simulink model "Avionics___Architecture_Model"  (R2022a)
settings: Solver=VariableStepAuto  StartTime=0.0  StopTime=10.0  RelTol=1e-3
settings Model: Creator=Kurt  LastModifiedBy=Kurt

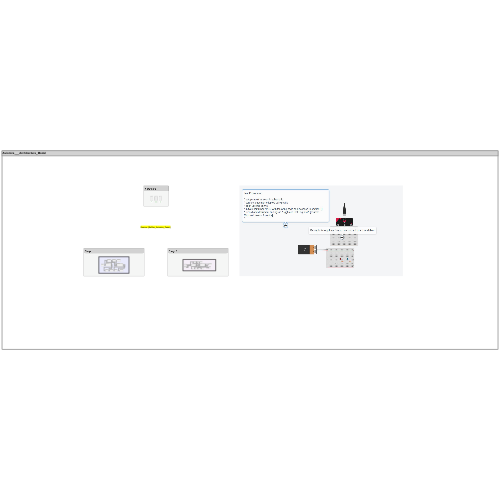
[thumbnail: Simulink's stored preview of the top-level diagram]
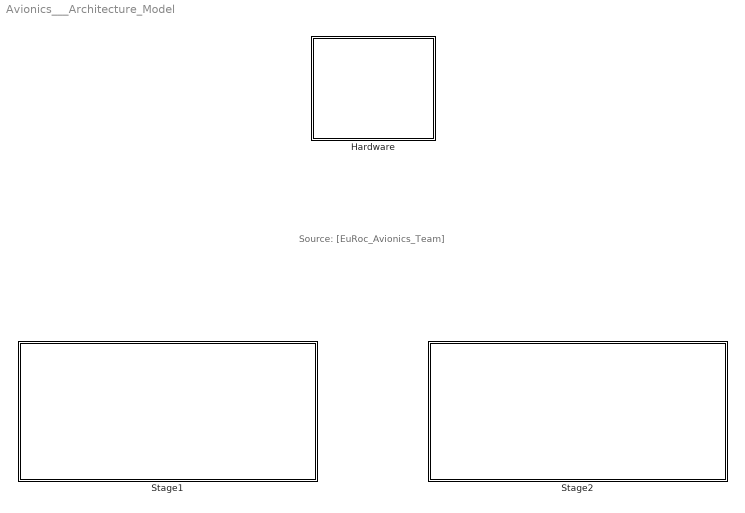
== system Avionics___Architecture_Model ==
  note: Source: [EuRoc_Avionics_Team]
  Hardware : Subsystem
      settings: PortSchema="{\"entries\":[{\"content\":{\"headerSize\":26,\"margin\":15,\"minimumSpacing\":25,\"sides\":[{\"content\":{\"connectorIds\":[]},\"type\":\"ConnectorPlacement.EquallySpacedRectSide\",\"uuid\":\"98d5147a-290e-4a67-98f4-450c53d1887a\"},{\"content\":{\"connectorIds\":[],\"side\":\"RIGHT\"},\"type\":\"ConnectorPlacement.EquallySpacedRectSide\",\"uuid\":\"a084b330-0c04-4420-9b8a-15d6db2d12b6\"},{\"content\":{\"connectorIds\":[],\"side\":\"TOP\"},\"type\":\"ConnectorPlacement.EquallySpacedRectSide\",\"uuid\":\"4cd23e2a-f423-4056-8b31-58661018ed01\"}]},\"type\":\"ConnectorPlacement.EquallySpacedConnector\",\"uuid\":\"58c578c1-1979-4184-bf96-9f147fef1420\"}],\"packageUris\":[\"http://schema.mathworks.com/mf0/Connector/R2020b\"],\"version\":\"1.0\"}"
  Stage1 : Subsystem
      settings: PortSchema="{\"entries\":[{\"content\":{\"headerSize\":26,\"margin\":15,\"minimumSpacing\":25,\"sides\":[{\"content\":{\"connectorIds\":[]},\"type\":\"ConnectorPlacement.EquallySpacedRectSide\",\"uuid\":\"98d5147a-290e-4a67-98f4-450c53d1887a\"},{\"content\":{\"connectorIds\":[],\"side\":\"RIGHT\"},\"type\":\"ConnectorPlacement.EquallySpacedRectSide\",\"uuid\":\"a084b330-0c04-4420-9b8a-15d6db2d12b6\"},{\"content\":{\"connectorIds\":[],\"side\":\"TOP\"},\"type\":\"ConnectorPlacement.EquallySpacedRectSide\",\"uuid\":\"4cd23e2a-f423-4056-8b31-58661018ed01\"}]},\"type\":\"ConnectorPlacement.EquallySpacedConnector\",\"uuid\":\"58c578c1-1979-4184-bf96-9f147fef1420\"}],\"packageUris\":[\"http://schema.mathworks.com/mf0/Connector/R2020b\"],\"version\":\"1.0\"}"
  Stage2 : Subsystem
      settings: PortSchema="{\"entries\":[{\"content\":{\"headerSize\":26,\"margin\":15,\"minimumSpacing\":25,\"sides\":[{\"content\":{\"connectorIds\":[]},\"type\":\"ConnectorPlacement.EquallySpacedRectSide\",\"uuid\":\"98d5147a-290e-4a67-98f4-450c53d1887a\"},{\"content\":{\"connectorIds\":[],\"side\":\"RIGHT\"},\"type\":\"ConnectorPlacement.EquallySpacedRectSide\",\"uuid\":\"a084b330-0c04-4420-9b8a-15d6db2d12b6\"},{\"content\":{\"connectorIds\":[],\"side\":\"TOP\"},\"type\":\"ConnectorPlacement.EquallySpacedRectSide\",\"uuid\":\"4cd23e2a-f423-4056-8b31-58661018ed01\"}]},\"type\":\"ConnectorPlacement.EquallySpacedConnector\",\"uuid\":\"58c578c1-1979-4184-bf96-9f147fef1420\"}],\"packageUris\":[\"http://schema.mathworks.com/mf0/Connector/R2020b\"],\"version\":\"1.0\"}"

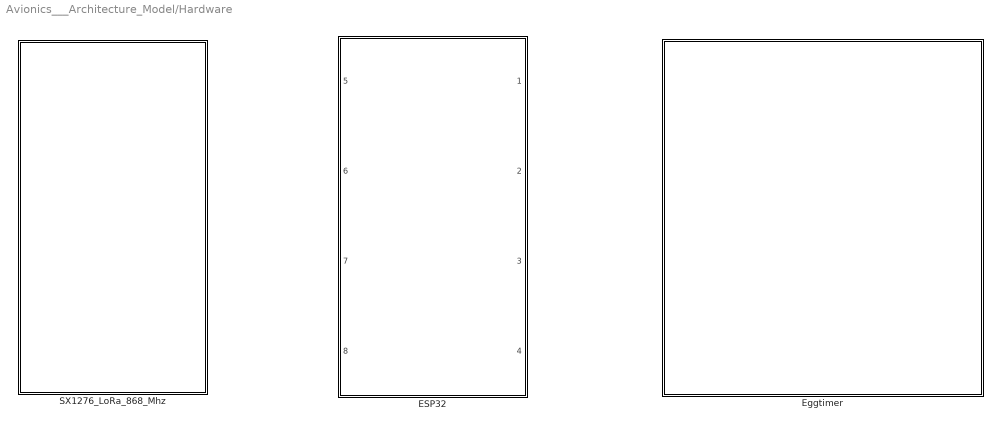
== system Avionics___Architecture_Model/Hardware ==
  ESP32 : Subsystem
      settings: PortSchema="{\"entries\":[{\"content\":{\"headerSize\":26,\"margin\":15,\"minimumSpacing\":25,\"sides\":[{\"content\":{\"connectorIds\":[\"In1\",\"In2\",\"In3\",\"In4\"]},\"type\":\"ConnectorPlacement.EquallySpacedRectSide\",\"uuid\":\"98d5147a-290e-4a67-98f4-450c53d1887a\"},{\"content\":{\"connectorIds\":[\"Out1\",\"Out2\",\"Out3\",\"Out4\"],\"side\":\"RIGHT\"},\"type\":\"ConnectorPlacement.EquallySpacedRectSide\",\"uuid\":\"a084b330-0c04-4420-9b8a-15d6db2d12b6\"},{\"content\":{\"connectorIds\":[],\"side\":\"TOP\"},\"type\":\"ConnectorPlacement.EquallySpacedRectSide\",\"uuid\":\"4cd23e2a-f423-4056-8b31-58661018ed01\"}]},\"type\":\"ConnectorPlacement.EquallySpacedConnector\",\"uuid\":\"58c578c1-1979-4184-bf96-9f147fef1420\"}],\"packageUris\":[\"http://schema.mathworks.com/mf0/Connector/R2020b\"],\"version\":\"1.0\"}"
  Eggtimer : Subsystem
      settings: PortSchema="{\"entries\":[{\"content\":{\"headerSize\":26,\"margin\":15,\"minimumSpacing\":25,\"sides\":[{\"content\":{\"connectorIds\":[\"LConn1\",\"LConn2\"]},\"type\":\"ConnectorPlacement.EquallySpacedRectSide\",\"uuid\":\"98d5147a-290e-4a67-98f4-450c53d1887a\"},{\"content\":{\"connectorIds\":[\"RConn1\",\"RConn2\",\"RConn3\",\"RConn4\"],\"side\":\"RIGHT\"},\"type\":\"ConnectorPlacement.EquallySpacedRectSide\",\"uuid\":\"a084b330-0c04-4420-9b8a-15d6db2d12b6\"},{\"content\":{\"connectorIds\":[\"LConn3\",\"LConn4\",\"LConn5\",\"LConn6\",\"LConn7\",\"LConn8\",\"LConn9\",\"LConn10\"],\"side\":\"TOP\"},\"type\":\"ConnectorPlacement.EquallySpacedRectSide\",\"uuid\":\"4cd23e2a-f423-4056-8b31-58661018ed01\"},{\"content\":{\"connectorIds\":[\"RConn5\",\"RConn6\",\"RConn7\",\"RConn8\",\"RConn9\",\"RConn10\"],\"side\":\"BOTTOM\"},\"type\":\"ConnectorPlacement.EquallySpacedRectSide\",\"uuid\":\"c712a256-adbb-4d26-ab18-9b9cb2ad7b77\"}]},\"type\":\"ConnectorPlacement.EquallySpacedConnector\",\"uuid\":\"58c578c1-1979-4184-bf96-9f147fef1420\"}],\"packageUris\":[\"http://schema.mathworks.com/mf0/Connector/R2020b\"],\"version\":\"1.0\"}"
  SX1276_LoRa_868_Mhz : Subsystem
      settings: PortSchema="{\"entries\":[{\"content\":{\"headerSize\":26,\"margin\":15,\"minimumSpacing\":25,\"sides\":[{\"content\":{\"connectorIds\":[]},\"type\":\"ConnectorPlacement.EquallySpacedRectSide\",\"uuid\":\"98d5147a-290e-4a67-98f4-450c53d1887a\"},{\"content\":{\"connectorIds\":[],\"side\":\"RIGHT\"},\"type\":\"ConnectorPlacement.EquallySpacedRectSide\",\"uuid\":\"a084b330-0c04-4420-9b8a-15d6db2d12b6\"},{\"content\":{\"connectorIds\":[],\"side\":\"TOP\"},\"type\":\"ConnectorPlacement.EquallySpacedRectSide\",\"uuid\":\"4cd23e2a-f423-4056-8b31-58661018ed01\"}]},\"type\":\"ConnectorPlacement.EquallySpacedConnector\",\"uuid\":\"58c578c1-1979-4184-bf96-9f147fef1420\"}],\"packageUris\":[\"http://schema.mathworks.com/mf0/Connector/R2020b\"],\"version\":\"1.0\"}"

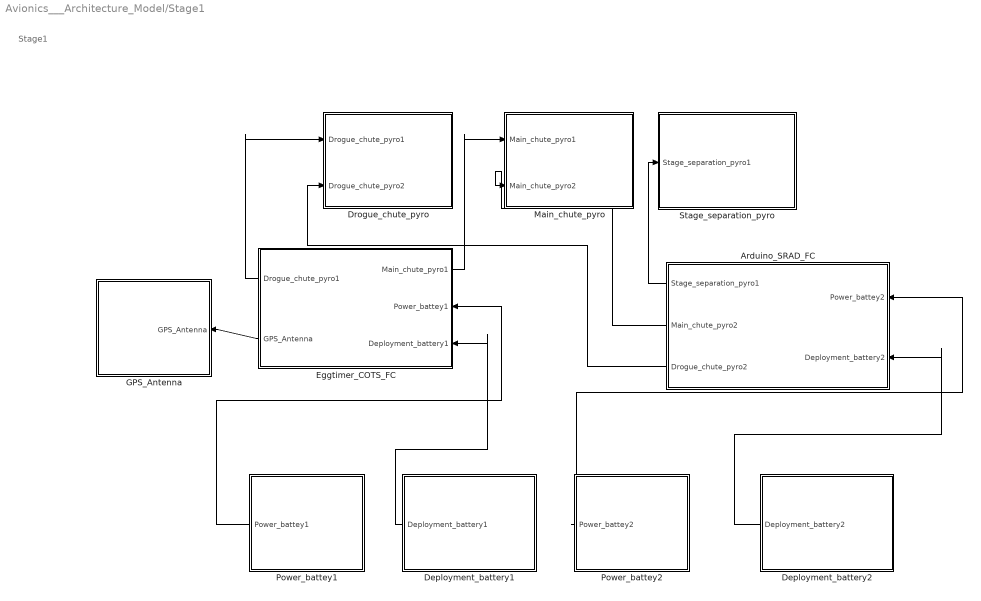
== system Avionics___Architecture_Model/Stage1 ==
  note: Stage1
  Arduino_SRAD_FC : Subsystem
      settings: PortSchema="{\"entries\":[{\"content\":{\"headerSize\":26,\"margin\":15,\"minimumSpacing\":25,\"sides\":[{\"content\":{\"connectorIds\":[\"Out1\",\"Out2\",\"Out3\"]},\"type\":\"ConnectorPlacement.EquallySpacedRectSide\",\"uuid\":\"98d5147a-290e-4a67-98f4-450c53d1887a\"},{\"content\":{\"connectorIds\":[\"In2\",\"In1\"],\"side\":\"RIGHT\"},\"type\":\"ConnectorPlacement.EquallySpacedRectSide\",\"uuid\":\"a084b330-0c04-4420-9b8a-15d6db2d12b6\"},{\"content\":{\"connectorIds\":[],\"side\":\"TOP\"},\"type\":\"ConnectorPlacement.EquallySpacedRectSide\",\"uuid\":\"4cd23e2a-f423-4056-8b31-58661018ed01\"},{\"content\":{\"connectorIds\":[],\"side\":\"BOTTOM\"},\"type\":\"ConnectorPlacement.EquallySpacedRectSide\",\"uuid\":\"eb863bb0-7cf9-4bf2-bc0b-ec6aafea4d0a\"}]},\"type\":\"ConnectorPlacement.EquallySpacedConnector\",\"uuid\":\"58c578c1-1979-4184-bf96-9f147fef1420\"}],\"packageUris\":[\"http://schema.mathworks.com/mf0/Connector/R2020b\"],\"version\":\"1.0\"}"
  Deployment_battery1 : Subsystem
      settings: PortSchema="{\"entries\":[{\"content\":{\"headerSize\":26,\"margin\":15,\"minimumSpacing\":25,\"sides\":[{\"content\":{\"connectorIds\":[\"Out1\"]},\"type\":\"ConnectorPlacement.EquallySpacedRectSide\",\"uuid\":\"98d5147a-290e-4a67-98f4-450c53d1887a\"},{\"content\":{\"connectorIds\":[],\"side\":\"RIGHT\"},\"type\":\"ConnectorPlacement.EquallySpacedRectSide\",\"uuid\":\"a084b330-0c04-4420-9b8a-15d6db2d12b6\"},{\"content\":{\"connectorIds\":[],\"side\":\"TOP\"},\"type\":\"ConnectorPlacement.EquallySpacedRectSide\",\"uuid\":\"4cd23e2a-f423-4056-8b31-58661018ed01\"}]},\"type\":\"ConnectorPlacement.EquallySpacedConnector\",\"uuid\":\"58c578c1-1979-4184-bf96-9f147fef1420\"}],\"packageUris\":[\"http://schema.mathworks.com/mf0/Connector/R2020b\"],\"version\":\"1.0\"}"
  Deployment_battery2 : Subsystem
      settings: PortSchema="{\"entries\":[{\"content\":{\"headerSize\":26,\"margin\":15,\"minimumSpacing\":25,\"sides\":[{\"content\":{\"connectorIds\":[\"Out1\"]},\"type\":\"ConnectorPlacement.EquallySpacedRectSide\",\"uuid\":\"98d5147a-290e-4a67-98f4-450c53d1887a\"},{\"content\":{\"connectorIds\":[],\"side\":\"RIGHT\"},\"type\":\"ConnectorPlacement.EquallySpacedRectSide\",\"uuid\":\"a084b330-0c04-4420-9b8a-15d6db2d12b6\"},{\"content\":{\"connectorIds\":[],\"side\":\"TOP\"},\"type\":\"ConnectorPlacement.EquallySpacedRectSide\",\"uuid\":\"4cd23e2a-f423-4056-8b31-58661018ed01\"}]},\"type\":\"ConnectorPlacement.EquallySpacedConnector\",\"uuid\":\"58c578c1-1979-4184-bf96-9f147fef1420\"}],\"packageUris\":[\"http://schema.mathworks.com/mf0/Connector/R2020b\"],\"version\":\"1.0\"}"
  Drogue_chute_pyro : Subsystem  Description=Reference: [Preliminary_CDR, CranSEDS,avionics team]
      settings: PortSchema="{\"entries\":[{\"content\":{\"headerSize\":26,\"margin\":15,\"minimumSpacing\":25,\"sides\":[{\"content\":{\"connectorIds\":[\"In1\",\"In2\"]},\"type\":\"ConnectorPlacement.EquallySpacedRectSide\",\"uuid\":\"98d5147a-290e-4a67-98f4-450c53d1887a\"},{\"content\":{\"connectorIds\":[],\"side\":\"RIGHT\"},\"type\":\"ConnectorPlacement.EquallySpacedRectSide\",\"uuid\":\"a084b330-0c04-4420-9b8a-15d6db2d12b6\"},{\"content\":{\"connectorIds\":[],\"side\":\"TOP\"},\"type\":\"ConnectorPlacement.EquallySpacedRectSide\",\"uuid\":\"4cd23e2a-f423-4056-8b31-58661018ed01\"}]},\"type\":\"ConnectorPlacement.EquallySpacedConnector\",\"uuid\":\"58c578c1-1979-4184-bf96-9f147fef1420\"}],\"packageUris\":[\"http://schema.mathworks.com/mf0/Connector/R2020b\"],\"version\":\"1.0\"}"
  Eggtimer_COTS_FC : Subsystem
      settings: PortSchema="{\"entries\":[{\"content\":{\"headerSize\":26,\"margin\":15,\"minimumSpacing\":25,\"sides\":[{\"content\":{\"connectorIds\":[\"Out2\",\"Out3\"]},\"type\":\"ConnectorPlacement.EquallySpacedRectSide\",\"uuid\":\"98d5147a-290e-4a67-98f4-450c53d1887a\"},{\"content\":{\"connectorIds\":[\"Out1\",\"In1\",\"In2\"],\"side\":\"RIGHT\"},\"type\":\"ConnectorPlacement.EquallySpacedRectSide\",\"uuid\":\"a084b330-0c04-4420-9b8a-15d6db2d12b6\"},{\"content\":{\"connectorIds\":[],\"side\":\"TOP\"},\"type\":\"ConnectorPlacement.EquallySpacedRectSide\",\"uuid\":\"4cd23e2a-f423-4056-8b31-58661018ed01\"}]},\"type\":\"ConnectorPlacement.EquallySpacedConnector\",\"uuid\":\"58c578c1-1979-4184-bf96-9f147fef1420\"}],\"packageUris\":[\"http://schema.mathworks.com/mf0/Connector/R2020b\"],\"version\":\"1.0\"}"
  GPS_Antenna : Subsystem
      settings: PortSchema="{\"entries\":[{\"content\":{\"headerSize\":26,\"margin\":15,\"minimumSpacing\":25,\"sides\":[{\"content\":{\"connectorIds\":[]},\"type\":\"ConnectorPlacement.EquallySpacedRectSide\",\"uuid\":\"98d5147a-290e-4a67-98f4-450c53d1887a\"},{\"content\":{\"connectorIds\":[\"In1\"],\"side\":\"RIGHT\"},\"type\":\"ConnectorPlacement.EquallySpacedRectSide\",\"uuid\":\"a084b330-0c04-4420-9b8a-15d6db2d12b6\"},{\"content\":{\"connectorIds\":[],\"side\":\"TOP\"},\"type\":\"ConnectorPlacement.EquallySpacedRectSide\",\"uuid\":\"4cd23e2a-f423-4056-8b31-58661018ed01\"}]},\"type\":\"ConnectorPlacement.EquallySpacedConnector\",\"uuid\":\"58c578c1-1979-4184-bf96-9f147fef1420\"}],\"packageUris\":[\"http://schema.mathworks.com/mf0/Connector/R2020b\"],\"version\":\"1.0\"}"
  Main_chute_pyro : Subsystem
      settings: PortSchema="{\"entries\":[{\"content\":{\"headerSize\":26,\"margin\":15,\"minimumSpacing\":25,\"sides\":[{\"content\":{\"connectorIds\":[\"In1\",\"In2\"]},\"type\":\"ConnectorPlacement.EquallySpacedRectSide\",\"uuid\":\"98d5147a-290e-4a67-98f4-450c53d1887a\"},{\"content\":{\"connectorIds\":[],\"side\":\"RIGHT\"},\"type\":\"ConnectorPlacement.EquallySpacedRectSide\",\"uuid\":\"a084b330-0c04-4420-9b8a-15d6db2d12b6\"},{\"content\":{\"connectorIds\":[],\"side\":\"TOP\"},\"type\":\"ConnectorPlacement.EquallySpacedRectSide\",\"uuid\":\"4cd23e2a-f423-4056-8b31-58661018ed01\"}]},\"type\":\"ConnectorPlacement.EquallySpacedConnector\",\"uuid\":\"58c578c1-1979-4184-bf96-9f147fef1420\"}],\"packageUris\":[\"http://schema.mathworks.com/mf0/Connector/R2020b\"],\"version\":\"1.0\"}"
  Power_battey1 : Subsystem
      settings: PortSchema="{\"entries\":[{\"content\":{\"headerSize\":26,\"margin\":15,\"minimumSpacing\":25,\"sides\":[{\"content\":{\"connectorIds\":[\"Out1\"]},\"type\":\"ConnectorPlacement.EquallySpacedRectSide\",\"uuid\":\"98d5147a-290e-4a67-98f4-450c53d1887a\"},{\"content\":{\"connectorIds\":[],\"side\":\"RIGHT\"},\"type\":\"ConnectorPlacement.EquallySpacedRectSide\",\"uuid\":\"a084b330-0c04-4420-9b8a-15d6db2d12b6\"},{\"content\":{\"connectorIds\":[],\"side\":\"TOP\"},\"type\":\"ConnectorPlacement.EquallySpacedRectSide\",\"uuid\":\"4cd23e2a-f423-4056-8b31-58661018ed01\"}]},\"type\":\"ConnectorPlacement.EquallySpacedConnector\",\"uuid\":\"58c578c1-1979-4184-bf96-9f147fef1420\"}],\"packageUris\":[\"http://schema.mathworks.com/mf0/Connector/R2020b\"],\"version\":\"1.0\"}"
  Power_battey2 : Subsystem
      settings: PortSchema="{\"entries\":[{\"content\":{\"headerSize\":26,\"margin\":15,\"minimumSpacing\":25,\"sides\":[{\"content\":{\"connectorIds\":[\"Out1\"]},\"type\":\"ConnectorPlacement.EquallySpacedRectSide\",\"uuid\":\"98d5147a-290e-4a67-98f4-450c53d1887a\"},{\"content\":{\"connectorIds\":[],\"side\":\"RIGHT\"},\"type\":\"ConnectorPlacement.EquallySpacedRectSide\",\"uuid\":\"a084b330-0c04-4420-9b8a-15d6db2d12b6\"},{\"content\":{\"connectorIds\":[],\"side\":\"TOP\"},\"type\":\"ConnectorPlacement.EquallySpacedRectSide\",\"uuid\":\"4cd23e2a-f423-4056-8b31-58661018ed01\"}]},\"type\":\"ConnectorPlacement.EquallySpacedConnector\",\"uuid\":\"58c578c1-1979-4184-bf96-9f147fef1420\"}],\"packageUris\":[\"http://schema.mathworks.com/mf0/Connector/R2020b\"],\"version\":\"1.0\"}"
  Stage_separation_pyro : Subsystem
      settings: PortSchema="{\"entries\":[{\"content\":{\"headerSize\":26,\"margin\":15,\"minimumSpacing\":25,\"sides\":[{\"content\":{\"connectorIds\":[\"In1\"]},\"type\":\"ConnectorPlacement.EquallySpacedRectSide\",\"uuid\":\"98d5147a-290e-4a67-98f4-450c53d1887a\"},{\"content\":{\"connectorIds\":[],\"side\":\"RIGHT\"},\"type\":\"ConnectorPlacement.EquallySpacedRectSide\",\"uuid\":\"a084b330-0c04-4420-9b8a-15d6db2d12b6\"},{\"content\":{\"connectorIds\":[],\"side\":\"TOP\"},\"type\":\"ConnectorPlacement.EquallySpacedRectSide\",\"uuid\":\"4cd23e2a-f423-4056-8b31-58661018ed01\"}]},\"type\":\"ConnectorPlacement.EquallySpacedConnector\",\"uuid\":\"58c578c1-1979-4184-bf96-9f147fef1420\"}],\"packageUris\":[\"http://schema.mathworks.com/mf0/Connector/R2020b\"],\"version\":\"1.0\"}"
  wires:
  Arduino_SRAD_FC/3(Drogue_chute_pyro2) -> Drogue_chute_pyro/2(Drogue_chute_pyro2)
  Deployment_battery1/1(Deployment_battery1) -> Eggtimer_COTS_FC/2(Deployment_battery1)
  Eggtimer_COTS_FC/2(Drogue_chute_pyro1) -> Drogue_chute_pyro/1(Drogue_chute_pyro1)
  Arduino_SRAD_FC/2(Main_chute_pyro2) -> Main_chute_pyro/2(Main_chute_pyro2)
  Eggtimer_COTS_FC/3(GPS_Antenna) -> GPS_Antenna/1(GPS_Antenna)
  Power_battey1/1(Power_battey1) -> Eggtimer_COTS_FC/1(Power_battey1)
  Eggtimer_COTS_FC/1(Main_chute_pyro1) -> Main_chute_pyro/1(Main_chute_pyro1)
  Arduino_SRAD_FC/1(Stage_separation_pyro1) -> Stage_separation_pyro/1(Stage_separation_pyro1)
  Deployment_battery2/1(Deployment_battery2) -> Arduino_SRAD_FC/1(Deployment_battery2)
  Power_battey2/1(Power_battey2) -> Arduino_SRAD_FC/2(Power_battey2)

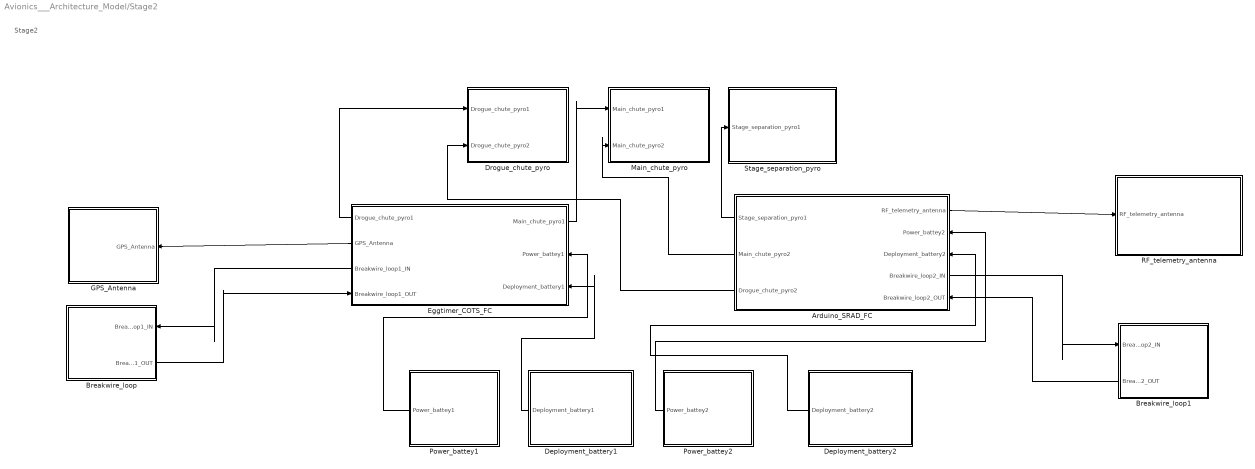
== system Avionics___Architecture_Model/Stage2 ==
  note: Stage2
  Arduino_SRAD_FC : Subsystem
      settings: PortSchema="{\"entries\":[{\"content\":{\"headerSize\":26,\"margin\":15,\"minimumSpacing\":25,\"sides\":[{\"content\":{\"connectorIds\":[\"Out3\",\"Out4\",\"Out5\"]},\"type\":\"ConnectorPlacement.EquallySpacedRectSide\",\"uuid\":\"98d5147a-290e-4a67-98f4-450c53d1887a\"},{\"content\":{\"connectorIds\":[\"Out1\",\"In2\",\"In1\",\"Out2\",\"In3\"],\"side\":\"RIGHT\"},\"type\":\"ConnectorPlacement.EquallySpacedRectSide\",\"uuid\":\"a084b330-0c04-4420-9b8a-15d6db2d12b6\"},{\"content\":{\"connectorIds\":[],\"side\":\"TOP\"},\"type\":\"ConnectorPlacement.EquallySpacedRectSide\",\"uuid\":\"4cd23e2a-f423-4056-8b31-58661018ed01\"},{\"content\":{\"connectorIds\":[],\"side\":\"BOTTOM\"},\"type\":\"ConnectorPlacement.EquallySpacedRectSide\",\"uuid\":\"eb863bb0-7cf9-4bf2-bc0b-ec6aafea4d0a\"}]},\"type\":\"ConnectorPlacement.EquallySpacedConnector\",\"uuid\":\"58c578c1-1979-4184-bf96-9f147fef1420\"}],\"packageUris\":[\"http://schema.mathworks.com/mf0/Connector/R2020b\"],\"version\":\"1.0\"}"
  Breakwire_loop : Subsystem
      settings: PortSchema="{\"entries\":[{\"content\":{\"headerSize\":26,\"margin\":15,\"minimumSpacing\":25,\"sides\":[{\"content\":{\"connectorIds\":[]},\"type\":\"ConnectorPlacement.EquallySpacedRectSide\",\"uuid\":\"98d5147a-290e-4a67-98f4-450c53d1887a\"},{\"content\":{\"connectorIds\":[\"In1\",\"Out1\"],\"side\":\"RIGHT\"},\"type\":\"ConnectorPlacement.EquallySpacedRectSide\",\"uuid\":\"a084b330-0c04-4420-9b8a-15d6db2d12b6\"},{\"content\":{\"connectorIds\":[],\"side\":\"TOP\"},\"type\":\"ConnectorPlacement.EquallySpacedRectSide\",\"uuid\":\"4cd23e2a-f423-4056-8b31-58661018ed01\"}]},\"type\":\"ConnectorPlacement.EquallySpacedConnector\",\"uuid\":\"58c578c1-1979-4184-bf96-9f147fef1420\"}],\"packageUris\":[\"http://schema.mathworks.com/mf0/Connector/R2020b\"],\"version\":\"1.0\"}"
  Breakwire_loop1 : Subsystem
      settings: PortSchema="{\"entries\":[{\"content\":{\"headerSize\":26,\"margin\":15,\"minimumSpacing\":25,\"sides\":[{\"content\":{\"connectorIds\":[\"In1\",\"Out1\"]},\"type\":\"ConnectorPlacement.EquallySpacedRectSide\",\"uuid\":\"98d5147a-290e-4a67-98f4-450c53d1887a\"},{\"content\":{\"connectorIds\":[],\"side\":\"RIGHT\"},\"type\":\"ConnectorPlacement.EquallySpacedRectSide\",\"uuid\":\"a084b330-0c04-4420-9b8a-15d6db2d12b6\"},{\"content\":{\"connectorIds\":[],\"side\":\"TOP\"},\"type\":\"ConnectorPlacement.EquallySpacedRectSide\",\"uuid\":\"4cd23e2a-f423-4056-8b31-58661018ed01\"}]},\"type\":\"ConnectorPlacement.EquallySpacedConnector\",\"uuid\":\"58c578c1-1979-4184-bf96-9f147fef1420\"}],\"packageUris\":[\"http://schema.mathworks.com/mf0/Connector/R2020b\"],\"version\":\"1.0\"}"
  Deployment_battery1 : Subsystem
      settings: PortSchema="{\"entries\":[{\"content\":{\"headerSize\":26,\"margin\":15,\"minimumSpacing\":25,\"sides\":[{\"content\":{\"connectorIds\":[\"Out1\"]},\"type\":\"ConnectorPlacement.EquallySpacedRectSide\",\"uuid\":\"98d5147a-290e-4a67-98f4-450c53d1887a\"},{\"content\":{\"connectorIds\":[],\"side\":\"RIGHT\"},\"type\":\"ConnectorPlacement.EquallySpacedRectSide\",\"uuid\":\"a084b330-0c04-4420-9b8a-15d6db2d12b6\"},{\"content\":{\"connectorIds\":[],\"side\":\"TOP\"},\"type\":\"ConnectorPlacement.EquallySpacedRectSide\",\"uuid\":\"4cd23e2a-f423-4056-8b31-58661018ed01\"}]},\"type\":\"ConnectorPlacement.EquallySpacedConnector\",\"uuid\":\"58c578c1-1979-4184-bf96-9f147fef1420\"}],\"packageUris\":[\"http://schema.mathworks.com/mf0/Connector/R2020b\"],\"version\":\"1.0\"}"
  Deployment_battery2 : Subsystem
      settings: PortSchema="{\"entries\":[{\"content\":{\"headerSize\":26,\"margin\":15,\"minimumSpacing\":25,\"sides\":[{\"content\":{\"connectorIds\":[\"Out1\"]},\"type\":\"ConnectorPlacement.EquallySpacedRectSide\",\"uuid\":\"98d5147a-290e-4a67-98f4-450c53d1887a\"},{\"content\":{\"connectorIds\":[],\"side\":\"RIGHT\"},\"type\":\"ConnectorPlacement.EquallySpacedRectSide\",\"uuid\":\"a084b330-0c04-4420-9b8a-15d6db2d12b6\"},{\"content\":{\"connectorIds\":[],\"side\":\"TOP\"},\"type\":\"ConnectorPlacement.EquallySpacedRectSide\",\"uuid\":\"4cd23e2a-f423-4056-8b31-58661018ed01\"}]},\"type\":\"ConnectorPlacement.EquallySpacedConnector\",\"uuid\":\"58c578c1-1979-4184-bf96-9f147fef1420\"}],\"packageUris\":[\"http://schema.mathworks.com/mf0/Connector/R2020b\"],\"version\":\"1.0\"}"
  Drogue_chute_pyro : Subsystem  Description=Reference: [Preliminary_CDR, CranSEDS,avionics team]
      settings: PortSchema="{\"entries\":[{\"content\":{\"headerSize\":26,\"margin\":15,\"minimumSpacing\":25,\"sides\":[{\"content\":{\"connectorIds\":[\"In1\",\"In2\"]},\"type\":\"ConnectorPlacement.EquallySpacedRectSide\",\"uuid\":\"98d5147a-290e-4a67-98f4-450c53d1887a\"},{\"content\":{\"connectorIds\":[],\"side\":\"RIGHT\"},\"type\":\"ConnectorPlacement.EquallySpacedRectSide\",\"uuid\":\"a084b330-0c04-4420-9b8a-15d6db2d12b6\"},{\"content\":{\"connectorIds\":[],\"side\":\"TOP\"},\"type\":\"ConnectorPlacement.EquallySpacedRectSide\",\"uuid\":\"4cd23e2a-f423-4056-8b31-58661018ed01\"}]},\"type\":\"ConnectorPlacement.EquallySpacedConnector\",\"uuid\":\"58c578c1-1979-4184-bf96-9f147fef1420\"}],\"packageUris\":[\"http://schema.mathworks.com/mf0/Connector/R2020b\"],\"version\":\"1.0\"}"
  Eggtimer_COTS_FC : Subsystem
      settings: PortSchema="{\"entries\":[{\"content\":{\"headerSize\":26,\"margin\":15,\"minimumSpacing\":25,\"sides\":[{\"content\":{\"connectorIds\":[\"Out2\",\"Out4\",\"Out3\",\"In1\"]},\"type\":\"ConnectorPlacement.EquallySpacedRectSide\",\"uuid\":\"98d5147a-290e-4a67-98f4-450c53d1887a\"},{\"content\":{\"connectorIds\":[\"Out1\",\"In2\",\"In3\"],\"side\":\"RIGHT\"},\"type\":\"ConnectorPlacement.EquallySpacedRectSide\",\"uuid\":\"a084b330-0c04-4420-9b8a-15d6db2d12b6\"},{\"content\":{\"connectorIds\":[],\"side\":\"TOP\"},\"type\":\"ConnectorPlacement.EquallySpacedRectSide\",\"uuid\":\"4cd23e2a-f423-4056-8b31-58661018ed01\"}]},\"type\":\"ConnectorPlacement.EquallySpacedConnector\",\"uuid\":\"58c578c1-1979-4184-bf96-9f147fef1420\"}],\"packageUris\":[\"http://schema.mathworks.com/mf0/Connector/R2020b\"],\"version\":\"1.0\"}"
  GPS_Antenna : Subsystem
      settings: PortSchema="{\"entries\":[{\"content\":{\"headerSize\":26,\"margin\":15,\"minimumSpacing\":25,\"sides\":[{\"content\":{\"connectorIds\":[]},\"type\":\"ConnectorPlacement.EquallySpacedRectSide\",\"uuid\":\"98d5147a-290e-4a67-98f4-450c53d1887a\"},{\"content\":{\"connectorIds\":[\"In1\"],\"side\":\"RIGHT\"},\"type\":\"ConnectorPlacement.EquallySpacedRectSide\",\"uuid\":\"a084b330-0c04-4420-9b8a-15d6db2d12b6\"},{\"content\":{\"connectorIds\":[],\"side\":\"TOP\"},\"type\":\"ConnectorPlacement.EquallySpacedRectSide\",\"uuid\":\"4cd23e2a-f423-4056-8b31-58661018ed01\"}]},\"type\":\"ConnectorPlacement.EquallySpacedConnector\",\"uuid\":\"58c578c1-1979-4184-bf96-9f147fef1420\"}],\"packageUris\":[\"http://schema.mathworks.com/mf0/Connector/R2020b\"],\"version\":\"1.0\"}"
  Main_chute_pyro : Subsystem
      settings: PortSchema="{\"entries\":[{\"content\":{\"headerSize\":26,\"margin\":15,\"minimumSpacing\":25,\"sides\":[{\"content\":{\"connectorIds\":[\"In1\",\"In2\"]},\"type\":\"ConnectorPlacement.EquallySpacedRectSide\",\"uuid\":\"98d5147a-290e-4a67-98f4-450c53d1887a\"},{\"content\":{\"connectorIds\":[],\"side\":\"RIGHT\"},\"type\":\"ConnectorPlacement.EquallySpacedRectSide\",\"uuid\":\"a084b330-0c04-4420-9b8a-15d6db2d12b6\"},{\"content\":{\"connectorIds\":[],\"side\":\"TOP\"},\"type\":\"ConnectorPlacement.EquallySpacedRectSide\",\"uuid\":\"4cd23e2a-f423-4056-8b31-58661018ed01\"}]},\"type\":\"ConnectorPlacement.EquallySpacedConnector\",\"uuid\":\"58c578c1-1979-4184-bf96-9f147fef1420\"}],\"packageUris\":[\"http://schema.mathworks.com/mf0/Connector/R2020b\"],\"version\":\"1.0\"}"
  Power_battey1 : Subsystem
      settings: PortSchema="{\"entries\":[{\"content\":{\"headerSize\":26,\"margin\":15,\"minimumSpacing\":25,\"sides\":[{\"content\":{\"connectorIds\":[\"Out1\"]},\"type\":\"ConnectorPlacement.EquallySpacedRectSide\",\"uuid\":\"98d5147a-290e-4a67-98f4-450c53d1887a\"},{\"content\":{\"connectorIds\":[],\"side\":\"RIGHT\"},\"type\":\"ConnectorPlacement.EquallySpacedRectSide\",\"uuid\":\"a084b330-0c04-4420-9b8a-15d6db2d12b6\"},{\"content\":{\"connectorIds\":[],\"side\":\"TOP\"},\"type\":\"ConnectorPlacement.EquallySpacedRectSide\",\"uuid\":\"4cd23e2a-f423-4056-8b31-58661018ed01\"}]},\"type\":\"ConnectorPlacement.EquallySpacedConnector\",\"uuid\":\"58c578c1-1979-4184-bf96-9f147fef1420\"}],\"packageUris\":[\"http://schema.mathworks.com/mf0/Connector/R2020b\"],\"version\":\"1.0\"}"
  Power_battey2 : Subsystem
      settings: PortSchema="{\"entries\":[{\"content\":{\"headerSize\":26,\"margin\":15,\"minimumSpacing\":25,\"sides\":[{\"content\":{\"connectorIds\":[\"Out1\"]},\"type\":\"ConnectorPlacement.EquallySpacedRectSide\",\"uuid\":\"98d5147a-290e-4a67-98f4-450c53d1887a\"},{\"content\":{\"connectorIds\":[],\"side\":\"RIGHT\"},\"type\":\"ConnectorPlacement.EquallySpacedRectSide\",\"uuid\":\"a084b330-0c04-4420-9b8a-15d6db2d12b6\"},{\"content\":{\"connectorIds\":[],\"side\":\"TOP\"},\"type\":\"ConnectorPlacement.EquallySpacedRectSide\",\"uuid\":\"4cd23e2a-f423-4056-8b31-58661018ed01\"}]},\"type\":\"ConnectorPlacement.EquallySpacedConnector\",\"uuid\":\"58c578c1-1979-4184-bf96-9f147fef1420\"}],\"packageUris\":[\"http://schema.mathworks.com/mf0/Connector/R2020b\"],\"version\":\"1.0\"}"
  RF_telemetry_antenna : Subsystem
      settings: PortSchema="{\"entries\":[{\"content\":{\"headerSize\":26,\"margin\":15,\"minimumSpacing\":25,\"sides\":[{\"content\":{\"connectorIds\":[\"In1\"]},\"type\":\"ConnectorPlacement.EquallySpacedRectSide\",\"uuid\":\"98d5147a-290e-4a67-98f4-450c53d1887a\"},{\"content\":{\"connectorIds\":[],\"side\":\"RIGHT\"},\"type\":\"ConnectorPlacement.EquallySpacedRectSide\",\"uuid\":\"a084b330-0c04-4420-9b8a-15d6db2d12b6\"},{\"content\":{\"connectorIds\":[],\"side\":\"TOP\"},\"type\":\"ConnectorPlacement.EquallySpacedRectSide\",\"uuid\":\"4cd23e2a-f423-4056-8b31-58661018ed01\"}]},\"type\":\"ConnectorPlacement.EquallySpacedConnector\",\"uuid\":\"58c578c1-1979-4184-bf96-9f147fef1420\"}],\"packageUris\":[\"http://schema.mathworks.com/mf0/Connector/R2020b\"],\"version\":\"1.0\"}"
  Stage_separation_pyro : Subsystem
      settings: PortSchema="{\"entries\":[{\"content\":{\"headerSize\":26,\"margin\":15,\"minimumSpacing\":25,\"sides\":[{\"content\":{\"connectorIds\":[\"In1\"]},\"type\":\"ConnectorPlacement.EquallySpacedRectSide\",\"uuid\":\"98d5147a-290e-4a67-98f4-450c53d1887a\"},{\"content\":{\"connectorIds\":[],\"side\":\"RIGHT\"},\"type\":\"ConnectorPlacement.EquallySpacedRectSide\",\"uuid\":\"a084b330-0c04-4420-9b8a-15d6db2d12b6\"},{\"content\":{\"connectorIds\":[],\"side\":\"TOP\"},\"type\":\"ConnectorPlacement.EquallySpacedRectSide\",\"uuid\":\"4cd23e2a-f423-4056-8b31-58661018ed01\"}]},\"type\":\"ConnectorPlacement.EquallySpacedConnector\",\"uuid\":\"58c578c1-1979-4184-bf96-9f147fef1420\"}],\"packageUris\":[\"http://schema.mathworks.com/mf0/Connector/R2020b\"],\"version\":\"1.0\"}"
  wires:
  Arduino_SRAD_FC/5(Drogue_chute_pyro2) -> Drogue_chute_pyro/2(Drogue_chute_pyro2)
  Deployment_battery1/1(Deployment_battery1) -> Eggtimer_COTS_FC/3(Deployment_battery1)
  Eggtimer_COTS_FC/2(Drogue_chute_pyro1) -> Drogue_chute_pyro/1(Drogue_chute_pyro1)
  Arduino_SRAD_FC/4(Main_chute_pyro2) -> Main_chute_pyro/2(Main_chute_pyro2)
  Eggtimer_COTS_FC/4(GPS_Antenna) -> GPS_Antenna/1(GPS_Antenna)
  Power_battey1/1(Power_battey1) -> Eggtimer_COTS_FC/2(Power_battey1)
  Eggtimer_COTS_FC/1(Main_chute_pyro1) -> Main_chute_pyro/1(Main_chute_pyro1)
  Arduino_SRAD_FC/3(Stage_separation_pyro1) -> Stage_separation_pyro/1(Stage_separation_pyro1)
  Deployment_battery2/1(Deployment_battery2) -> Arduino_SRAD_FC/1(Deployment_battery2)
  Power_battey2/1(Power_battey2) -> Arduino_SRAD_FC/2(Power_battey2)
  Eggtimer_COTS_FC/3(Breakwire_loop1_IN) -> Breakwire_loop/1(Breakwire_loop1_IN)
  Breakwire_loop/1(Breakwire_loop1_OUT) -> Eggtimer_COTS_FC/1(Breakwire_loop1_OUT)
  Arduino_SRAD_FC/1(RF_telemetry_antenna) -> RF_telemetry_antenna/1(RF_telemetry_antenna)
  Arduino_SRAD_FC/2(Breakwire_loop2_IN) -> Breakwire_loop1/1(Breakwire_loop2_IN)
  Breakwire_loop1/1(Breakwire_loop2_OUT) -> Arduino_SRAD_FC/3(Breakwire_loop2_OUT)

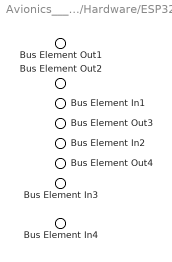
== system Avionics___Architecture_Model/Hardware/ESP32 ==
  Bus Element In1 : Inport  PortName=5
  Bus Element In2 : Inport  Port=2  PortName=6
  Bus Element In3 : Inport  Port=3  PortName=7
  Bus Element In4 : Inport  Port=4  PortName=8
  Bus Element Out1 : Outport  PortName=1
  Bus Element Out2 : Outport  Port=2  PortName=2
  Bus Element Out3 : Outport  Port=3  PortName=3
  Bus Element Out4 : Outport  Port=4  PortName=4

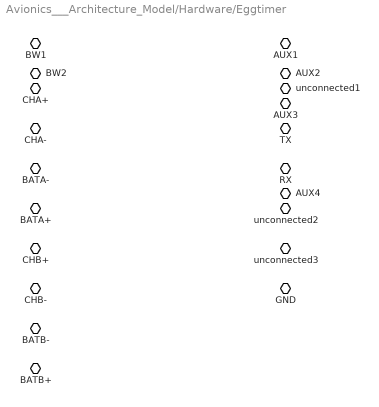
== system Avionics___Architecture_Model/Hardware/Eggtimer ==
  BW1 : PMIOPort  Side=Left
  BW2 : PMIOPort  Port=2  Side=Left
  CHA+ : PMIOPort  Port=3  Side=Left
  CHA- : PMIOPort  Port=4  Side=Left
  BATA- : PMIOPort  Port=5  Side=Left
  BATA+ : PMIOPort  Port=6  Side=Left
  CHB+ : PMIOPort  Port=7  Side=Left
  CHB- : PMIOPort  Port=8  Side=Left
  BATB- : PMIOPort  Port=9  Side=Left
  BATB+ : PMIOPort  Port=10  Side=Left
  AUX1 : PMIOPort  Port=11  Side=Right
  AUX2 : PMIOPort  Port=12  Side=Right
  AUX3 : PMIOPort  Port=13  Side=Right
  AUX4 : PMIOPort  Port=14  Side=Right
  unconnected1 : PMIOPort  Port=15  Side=Right
  TX : PMIOPort  Port=16  Side=Right
  RX : PMIOPort  Port=17  Side=Right
  unconnected2 : PMIOPort  Port=18  Side=Right
  unconnected3 : PMIOPort  Port=19  Side=Right
  GND : PMIOPort  Port=20  Side=Right

== system Avionics___Architecture_Model/Hardware/SX1276_LoRa_868_Mhz ==

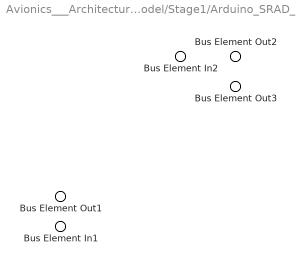
== system Avionics___Architecture_Model/Stage1/Arduino_SRAD_FC ==
  Bus Element In2 : Inport  PortName=Deployment_battery2
  Bus Element In1 : Inport  Port=2  PortName=Power_battey2
  Bus Element Out3 : Outport  PortName=Stage_separation_pyro1
  Bus Element Out2 : Outport  Port=2  PortName=Main_chute_pyro2
  Bus Element Out1 : Outport  Port=3  PortName=Drogue_chute_pyro2

== system Avionics___Architecture_Model/Stage1/Deployment_battery1 ==
  Bus Element Out1 : Outport  PortName=Deployment_battery1

== system Avionics___Architecture_Model/Stage1/Deployment_battery2 ==
  Bus Element Out1 : Outport  PortName=Deployment_battery2

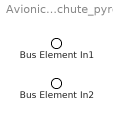
== system Avionics___Architecture_Model/Stage1/Drogue_chute_pyro ==
  Bus Element In1 : Inport  PortName=Drogue_chute_pyro1
  Bus Element In2 : Inport  Port=2  PortName=Drogue_chute_pyro2

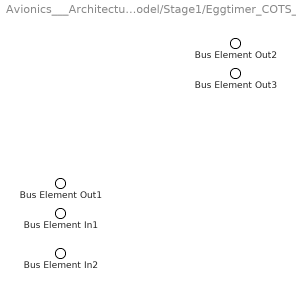
== system Avionics___Architecture_Model/Stage1/Eggtimer_COTS_FC ==
  Bus Element In1 : Inport  PortName=Power_battey1
  Bus Element In2 : Inport  Port=2  PortName=Deployment_battery1
  Bus Element Out3 : Outport  PortName=Main_chute_pyro1
  Bus Element Out2 : Outport  Port=2  PortName=Drogue_chute_pyro1
  Bus Element Out1 : Outport  Port=3  PortName=GPS_Antenna

== system Avionics___Architecture_Model/Stage1/GPS_Antenna ==
  Bus Element In1 : Inport  PortName=GPS_Antenna

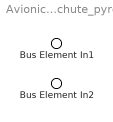
== system Avionics___Architecture_Model/Stage1/Main_chute_pyro ==
  Bus Element In1 : Inport  PortName=Main_chute_pyro1
  Bus Element In2 : Inport  Port=2  PortName=Main_chute_pyro2

== system Avionics___Architecture_Model/Stage1/Power_battey1 ==
  Bus Element Out1 : Outport  PortName=Power_battey1

== system Avionics___Architecture_Model/Stage1/Power_battey2 ==
  Bus Element Out1 : Outport  PortName=Power_battey2

== system Avionics___Architecture_Model/Stage1/Stage_separation_pyro ==
  Bus Element In1 : Inport  PortName=Stage_separation_pyro1

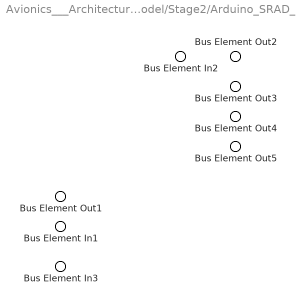
== system Avionics___Architecture_Model/Stage2/Arduino_SRAD_FC ==
  Bus Element In2 : Inport  PortName=Deployment_battery2
  Bus Element In1 : Inport  Port=2  PortName=Power_battey2
  Bus Element In3 : Inport  Port=3  PortName=Breakwire_loop2_OUT
  Bus Element Out4 : Outport  PortName=RF_telemetry_antenna
  Bus Element Out5 : Outport  Port=2  PortName=Breakwire_loop2_IN
  Bus Element Out3 : Outport  Port=3  PortName=Stage_separation_pyro1
  Bus Element Out2 : Outport  Port=4  PortName=Main_chute_pyro2
  Bus Element Out1 : Outport  Port=5  PortName=Drogue_chute_pyro2

== system Avionics___Architecture_Model/Stage2/Breakwire_loop ==
  Bus Element In1 : Inport  PortName=Breakwire_loop1_IN
  Bus Element Out1 : Outport  PortName=Breakwire_loop1_OUT

== system Avionics___Architecture_Model/Stage2/Breakwire_loop1 ==
  Bus Element In1 : Inport  PortName=Breakwire_loop2_IN
  Bus Element Out1 : Outport  PortName=Breakwire_loop2_OUT

== system Avionics___Architecture_Model/Stage2/Deployment_battery1 ==
  Bus Element Out1 : Outport  PortName=Deployment_battery1

== system Avionics___Architecture_Model/Stage2/Deployment_battery2 ==
  Bus Element Out1 : Outport  PortName=Deployment_battery2

== system Avionics___Architecture_Model/Stage2/Drogue_chute_pyro ==
  Bus Element In1 : Inport  PortName=Drogue_chute_pyro1
  Bus Element In2 : Inport  Port=2  PortName=Drogue_chute_pyro2

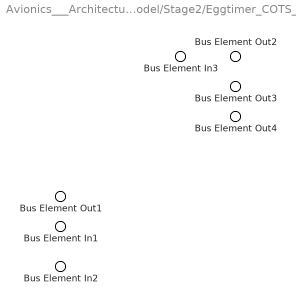
== system Avionics___Architecture_Model/Stage2/Eggtimer_COTS_FC ==
  Bus Element In3 : Inport  PortName=Breakwire_loop1_OUT
  Bus Element In1 : Inport  Port=2  PortName=Power_battey1
  Bus Element In2 : Inport  Port=3  PortName=Deployment_battery1
  Bus Element Out3 : Outport  PortName=Main_chute_pyro1
  Bus Element Out2 : Outport  Port=2  PortName=Drogue_chute_pyro1
  Bus Element Out4 : Outport  Port=3  PortName=Breakwire_loop1_IN
  Bus Element Out1 : Outport  Port=4  PortName=GPS_Antenna

== system Avionics___Architecture_Model/Stage2/GPS_Antenna ==
  Bus Element In1 : Inport  PortName=GPS_Antenna

== system Avionics___Architecture_Model/Stage2/Main_chute_pyro ==
  Bus Element In1 : Inport  PortName=Main_chute_pyro1
  Bus Element In2 : Inport  Port=2  PortName=Main_chute_pyro2

== system Avionics___Architecture_Model/Stage2/Power_battey1 ==
  Bus Element Out1 : Outport  PortName=Power_battey1

== system Avionics___Architecture_Model/Stage2/Power_battey2 ==
  Bus Element Out1 : Outport  PortName=Power_battey2

== system Avionics___Architecture_Model/Stage2/RF_telemetry_antenna ==
  Bus Element In1 : Inport  PortName=RF_telemetry_antenna

== system Avionics___Architecture_Model/Stage2/Stage_separation_pyro ==
  Bus Element In1 : Inport  PortName=Stage_separation_pyro1
